simulink model "Exp3_Simulink1"  (R2018b)
settings: Solver=VariableStepAuto  StartTime=0.0  StopTime=50  RelTol=1e-3
libraries: simulink x1
settings Model: Creator=Administrator  LastModifiedBy=Administrator

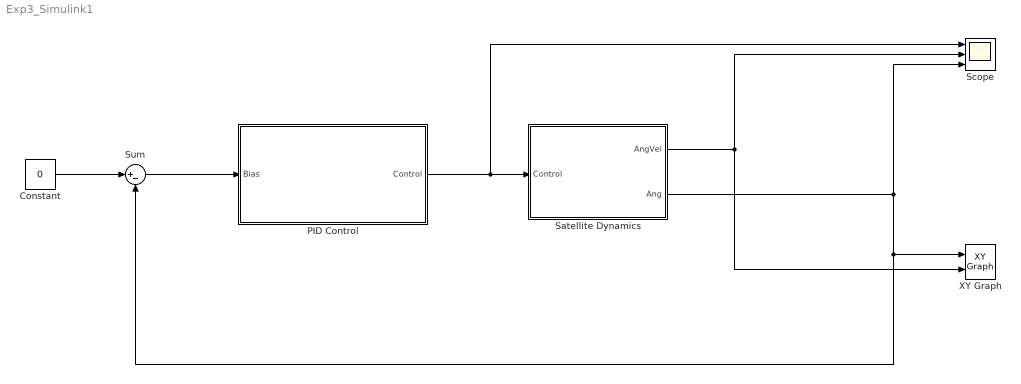
== system Exp3_Simulink1 ==
  Constant : Constant  Value=0
  PID Control : Subsystem  mask(注意){kp=2, ki=0, kd=10}
      mask prompts: kp "控制参数kp"; ki "控制参数ki"; kd "控制参数kd"
      mask help: 此模块为封装好的PID控制模块，可以自行设置PID参数
      mask Help: 哈工大版权所有
  Satellite Dynamics : Subsystem
  Scope : Scope  NumInputPorts=3
  Sum : Sum  Inputs=|+-
  XY Graph : simulink/Sinks/XY Graph  xmin=-1  xmax=1  ymin=-1  ymax=1  st=-1
  wires:
  Constant/1 -> Sum/1
  PID Control/1(Control) -> Scope/1, Satellite Dynamics/1(Control)
  Sum/1 -> PID Control/1(Bias)
  Satellite Dynamics/1(AngVel) -> XY Graph/2, Scope/2
  Satellite Dynamics/2(Ang) -> XY Graph/1, Sum/2, Scope/3

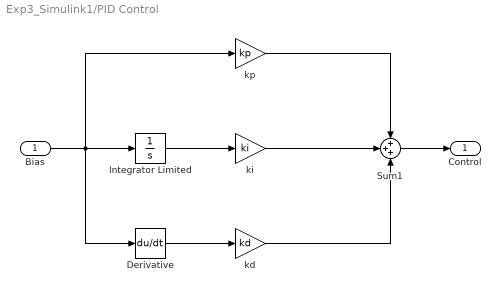
== system Exp3_Simulink1/PID Control ==
  Bias : Inport
  Derivative : Derivative
  Integrator Limited : Integrator  LimitOutput=on  UpperSaturationLimit=0.05  LowerSaturationLimit=-0.05
  Sum1 : Sum  Inputs=+++
  kd : Gain  Gain=kd
  ki : Gain  Gain=ki
  kp : Gain  Gain=kp
  Control : Outport
  wires:
  Derivative/1 -> kd/1
  Integrator Limited/1 -> ki/1
  kd/1 -> Sum1/3
  Bias/1 -> Integrator Limited/1, kp/1, Derivative/1
  Sum1/1 -> Control/1
  kp/1 -> Sum1/1
  ki/1 -> Sum1/2

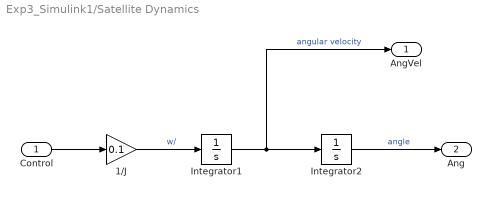
== system Exp3_Simulink1/Satellite Dynamics ==
  Control : Inport
  1/J : Gain  Gain=0.1
  Integrator1 : Integrator  InitialCondition=-0.5
  Integrator2 : Integrator  InitialCondition=1
  AngVel : Outport
  Ang : Outport  Port=2
  wires:
  1/J/1 -> Integrator1/1  "w/"
  Control/1 -> 1/J/1
  Integrator1/1 -> Integrator2/1, AngVel/1  "angular velocity"
  Integrator2/1 -> Ang/1  "angle"
